simulink model "new"  (R2020a)
settings: Solver=VariableStepAuto  StartTime=0.0  StopTime=3.0  RelTol=1e-3
libraries: dsparch4 x1
settings Model: Creator=dinhm  LastModifiedBy=dinhm

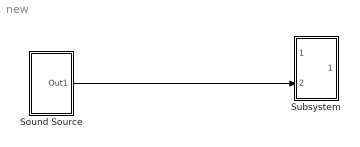
== system new ==
  Sound Source : Subsystem
  Subsystem : Subsystem
  wires:
  Sound Source/1(Out1) -> Subsystem/2(In2)

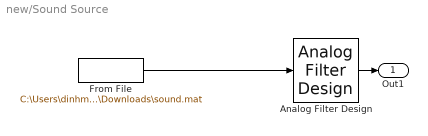
== system new/Sound Source ==
  Analog Filter Design : dsparch4/Analog Filter Design  method=Butterworth  filttype=Lowpass  N=8  Wlo=2*pi*4e3  Whi=80  Rp=2  Rs=40
  From File : FromFile  FileName=C:\Users\dinhm\Downloads\sound.mat  SampleTime=0
  Out1 : Outport
  wires:
  From File/1 -> Analog Filter Design/1
  Analog Filter Design/1 -> Out1/1

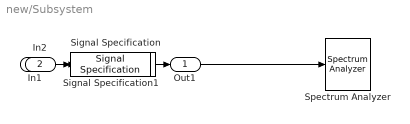
== system new/Subsystem ==
  In1 : Inport
  In2 : Inport  Port=2
  Signal Specification : SignalSpecification  SampleTime=1/16e4
  Signal Specification1 : SignalSpecification  SampleTime=1/16e4
  Spectrum Analyzer : SpectrumAnalyzer
  Out1 : Outport
  wires:
  Signal Specification/1 -> Spectrum Analyzer/1
  In2/1 -> Signal Specification/1
  In1/1 -> Signal Specification1/1
  Signal Specification1/1 -> Out1/1
